simulink model "Deadbeat_Sim"  (R2018b)
settings: Solver=VariableStepAuto  StartTime=0.0  StopTime=0.5  MaxStep=1E-6  RelTol=1E-5
values from neighbouring files (symbols this model uses):
  K0 = -2.5    [Deadbeat.m]
  K1 = [1.3018 0.0001]    [Deadbeat.m]    (also in Deadbeat2.m = Kr(1, 1:2))
  L = K'    [Deadbeat.m]    (also in Deadbeat2.m = Q*[b0-a0; b1-a1])
undefined symbols (not defined in the file or in its folder): A, B, C
settings Model: Creator=Biao Cheng  LastModifiedBy=ohara

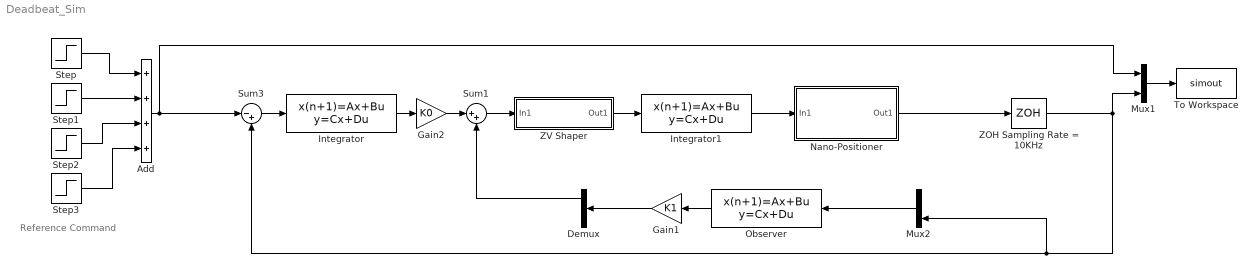
== system Deadbeat_Sim ==
  note: Reference Command
  Add : Sum  Inputs=++++
  Demux : Demux  Outputs=2
  Gain1 : Gain  Gain=K1
  Gain2 : Gain  Gain=K0
  Integrator : DiscreteStateSpace  C=.59  D=0  SampleTime=1E-4
  Integrator1 : DiscreteStateSpace  A=.49  B=.4  C=.67  D=0  SampleTime=1E-4
  Mux1 : Mux  Inputs=2
  Mux2 : Mux  Inputs=2
  Nano-Positioner : Subsystem
  "Observer " : DiscreteStateSpace  A=A-L*C  B=[B L]  C=[1 0 0; 0 0 1]  D=[0 0; 0 0]  SampleTime=1E-4
  Step : Step  Time=5E-3  SampleTime=0
  Step1 : Step  Time=15E-3  SampleTime=0
  Step2 : Step  Time=25E-3  After=-1  SampleTime=0
  Step3 : Step  Time=35E-3  After=-1  SampleTime=0
  Sum1 : Sum  Inputs=|++
  Sum3 : Sum  Inputs=|-+  AccumDataTypeStr=double
  To Workspace : ToWorkspace  VariableName=simout  SaveFormat=Timeseries  SampleTime=1/10000
  ZOH Sampling Rate = 10KHz : ZeroOrderHold  SampleTime=1E-5
  "ZV Shaper " : Subsystem
  wires:
  Step/1 -> Add/1
  Step1/1 -> Add/2
  Step2/1 -> Add/3
  Step3/1 -> Add/4
  "Observer "/1 -> Gain1/1
  Nano-Positioner/1(Out1) -> ZOH Sampling Rate = 10KHz/1
  ZOH Sampling Rate = 10KHz/1 -> Mux1/2, Sum3/2, Mux2/2
  Integrator/1 -> Gain2/1
  Add/1 -> Sum3/1, Mux1/1
  Sum1/1 -> "ZV Shaper "/1(In1)
  Demux/1 -> Sum1/2
  Mux1/1 -> To Workspace/1
  Gain2/1 -> Sum1/1
  Sum3/1 -> Integrator/1
  Gain1/1 -> Demux/1
  Mux2/1 -> "Observer "/1
  Integrator1/1 -> Nano-Positioner/1(In1)
  "ZV Shaper "/1(Out1) -> Integrator1/1

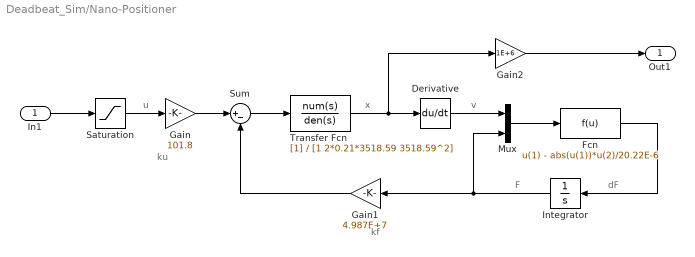
== system Deadbeat_Sim/Nano-Positioner ==
  note: dF
  note: F
  note: v
  note: x
  note: kf
  note: u
  note: ku
  In1 : Inport
  Derivative : Derivative
  Fcn : Fcn  Expr=u(1) - abs(u(1))*u(2)/20.22E-6
  Gain : Gain  Gain=101.8
  Gain1 : Gain  Gain=4.987E+7
  Gain2 : Gain  Gain=1E+6
  Integrator : Integrator
  Mux : Mux  Inputs=2
  Saturation : Saturate  UpperLimit=4  LowerLimit=-4
  Sum : Sum  Inputs=|+-
  Transfer Fcn : TransferFcn  Denominator=[1 2*0.21*3518.59 3518.59^2]
  Out1 : Outport
  wires:
  Gain1/1 -> Sum/2
  Mux/1 -> Fcn/1
  Integrator/1 -> Mux/2, Gain1/1
  In1/1 -> Saturation/1
  Derivative/1 -> Mux/1
  Fcn/1 -> Integrator/1
  Sum/1 -> Transfer Fcn/1
  Saturation/1 -> Gain/1
  Gain/1 -> Sum/1
  Transfer Fcn/1 -> Gain2/1, Derivative/1
  Gain2/1 -> Out1/1

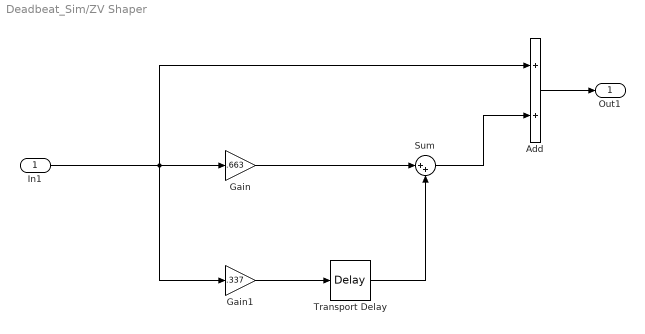
== system Deadbeat_Sim/ZV Shaper  ==
  In1 : Inport
  Add : Sum
  Gain : Gain  Gain=.663
  Gain1 : Gain  Gain=.337
  Sum : Sum  Inputs=|++
  Transport Delay : TransportDelay  DelayTime=1E-3
  Out1 : Outport
  wires:
  Gain1/1 -> Transport Delay/1
  Transport Delay/1 -> Sum/2
  Gain/1 -> Sum/1
  Sum/1 -> Add/2
  Add/1 -> Out1/1
  In1/1 -> Add/1, Gain1/1, Gain/1
